simulink model "simc"  (R2020b)
settings: Solver=ode45  StartTime=0.0  StopTime=0.0005  RelTol=1e-3
values from neighbouring files (symbols this model uses):
  A = 8    [iraep.m]
  C = 9.5812e-5    (= 9.5812e-05)    [iraep.m]
  k = 1/(10^(-8.41/20))    (= 2.63329794368)    [iraep.m]
  ku1 = 0.7468    [iraep.m]
  L = 5.0498e-5    (= 5.0498e-05)    [iraep.m]
  Rs = 2.66    [iraep.m]    (also in simulare.m)
  U21 = 16    [iraep.m]
undefined symbols (not defined in the file or in its folder): den_pi, num_pi
settings Model: Creator=Alex  LastModifiedBy=Alex

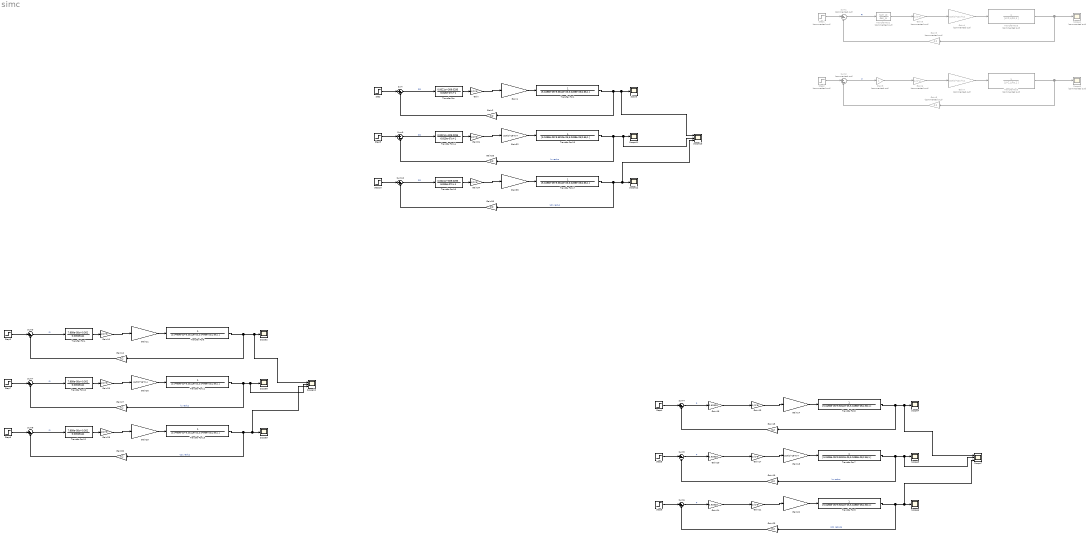
== system simc ==
  Gain{,10,13,17,21,25,28,31,34} (9 alike) : Gain  Gain=1/(2*8)
  Gain1 : Gain  Gain=sqrt(2)*16*0.7468
  Gain11 : Gain  Gain=sqrt(2)*16*0.7468
  Gain{2,12,15,19,23,27,30,33,36} (9 alike) : Gain  Gain=0.2
  Gain14 : Gain  Gain=sqrt(2)*16*0.7468
  Gain16 : Gain  Gain=2.63329
  Gain18 : Gain  Gain=sqrt(2)*16*0.4
  Gain20 : Gain  Gain=2.63329
  Gain22 : Gain  Gain=sqrt(2)*13*0.7468
  Gain24 : Gain  Gain=2.63329
  Gain26 : Gain  Gain=sqrt(2)*16*0.4
  Gain29 : Gain  Gain=sqrt(2)*13*0.7468
  Gain3 : Gain  Commented=on  Gain=1/(2*A)
  Gain32 : Gain  Gain=sqrt(2)*16*0.4
  Gain35 : Gain  Gain=sqrt(2)*13*0.7468
  Gain4 : Gain  Commented=on  Gain=sqrt(2)*U21*ku1
  Gain5 : Gain  Commented=on  Gain=0.2
  Gain6 : Gain  Commented=on  Gain=1/(2*A)
  Gain7 : Gain  Commented=on  Gain=sqrt(2)*U21*ku1
  Gain8 : Gain  Commented=on  Gain=0.2
  Gain9 : Gain  Commented=on  Gain=k
  Scope{,2,4..6,8..9,11..12} (9 alike) : Scope
  Scope1 : Scope  Commented=on
  Scope10 : Scope  NumInputPorts=3
  Scope13 : Scope  NumInputPorts=3
  Scope3 : Scope  Commented=on
  Scope7 : Scope  NumInputPorts=3
  Step{,3..10} (9 alike) : Step  Time=0  After=1.6  SampleTime=0
  Step1 : Step  Commented=on  Time=0  SampleTime=0
  Step2 : Step  Commented=on  Time=0  SampleTime=0
  Sum{,3..10} (9 alike) : Sum  Inputs=|+-
  Sum1 : Sum  Commented=on  Inputs=|+-
  Sum2 : Sum  Commented=on  Inputs=|+-
  Transfer Fcn : TransferFcn  Numerator="[0.0021  309.0295]"  Denominator=[6.815e-07 1]
  Transfer Fcn{1,6..9,11,13,15,17} (9 alike) : TransferFcn  Denominator=[5.0498e-05*9.5812e-05,5.0498e-05/2.66,1 ]
  Transfer Fcn10 : TransferFcn  Numerator="[7.895e-05  0.302]"  Denominator=[0.0002614 0]
  Transfer Fcn12 : TransferFcn  Numerator="[7.895e-05  0.302]"  Denominator=[0.0002614 0]
  Transfer Fcn14 : TransferFcn  Numerator="[0.0021  309.0295]"  Denominator=[6.815e-07 1]
  Transfer Fcn16 : TransferFcn  Numerator="[0.0021  309.0295]"  Denominator=[6.815e-07 1]
  Transfer Fcn2 : TransferFcn  Commented=on  Numerator=num_pi  Denominator=den_pi
  Transfer Fcn3 : TransferFcn  Commented=on  Denominator=[L*C,L/Rs,1 ]
  Transfer Fcn4 : TransferFcn  Numerator="[7.895e-05  0.302]"  Denominator=[0.0002614 0]
  Transfer Fcn5 : TransferFcn  Commented=on  Denominator=[L*C,L/Rs,1 ]
  wires:
  Step/1 -> Sum/1
  Sum/1 -> Transfer Fcn/1  "PD"
  Transfer Fcn/1 -> Gain/1
  Gain/1 -> Gain1/1
  Gain1/1 -> Transfer Fcn1/1
  Transfer Fcn1/1 -> Gain2/1, Scope13/1, Scope/1
  Gain2/1 -> Sum/2
  Gain5/1 -> Sum1/2
  Transfer Fcn3/1 -> Gain5/1, Scope1/1
  Gain4/1 -> Transfer Fcn3/1
  Gain3/1 -> Gain4/1
  Transfer Fcn2/1 -> Gain3/1
  Sum1/1 -> Transfer Fcn2/1  "PI"
  Step1/1 -> Sum1/1
  Step2/1 -> Sum2/1
  Sum2/1 -> Gain9/1  "P"
  Gain9/1 -> Gain6/1
  Gain6/1 -> Gain7/1
  Gain7/1 -> Transfer Fcn5/1
  Transfer Fcn5/1 -> Scope3/1, Gain8/1
  Gain8/1 -> Sum2/2
  Gain12/1 -> Sum3/2
  Transfer Fcn6/1 -> Scope10/1, Scope2/1, Gain12/1
  Gain11/1 -> Transfer Fcn6/1
  Gain10/1 -> Gain11/1
  Transfer Fcn4/1 -> Gain10/1
  Sum3/1 -> Transfer Fcn4/1  "PI"
  Step3/1 -> Sum3/1
  Step4/1 -> Sum4/1
  Sum4/1 -> Gain16/1  "P"
  Gain16/1 -> Gain13/1
  Gain13/1 -> Gain14/1
  Gain14/1 -> Transfer Fcn8/1
  Transfer Fcn8/1 -> Gain15/1, Scope7/1, Scope4/1
  Gain15/1 -> Sum4/2
  Gain19/1 -> Sum5/2
  Transfer Fcn7/1 -> Scope7/2, Scope5/1, Gain19/1  "ku redus"
  Gain18/1 -> Transfer Fcn7/1
  Gain17/1 -> Gain18/1
  Gain20/1 -> Gain17/1
  Sum5/1 -> Gain20/1  "P"
  Step5/1 -> Sum5/1
  Step6/1 -> Sum6/1
  Sum6/1 -> Gain24/1  "P"
  Gain24/1 -> Gain21/1
  Gain21/1 -> Gain22/1
  Gain22/1 -> Transfer Fcn9/1
  Transfer Fcn9/1 -> Gain23/1, Scope7/3, Scope6/1  "U21 redusa"
  Gain23/1 -> Sum6/2
  Step7/1 -> Sum7/1
  Sum7/1 -> Transfer Fcn10/1  "PI"
  Transfer Fcn10/1 -> Gain25/1
  Gain25/1 -> Gain26/1
  Gain26/1 -> Transfer Fcn11/1
  Transfer Fcn11/1 -> Gain27/1, Scope10/2, Scope8/1  "ku redus"
  Gain27/1 -> Sum7/2
  Gain30/1 -> Sum8/2
  Transfer Fcn13/1 -> Scope10/3, Scope9/1, Gain30/1  "U21 redus"
  Gain29/1 -> Transfer Fcn13/1
  Gain28/1 -> Gain29/1
  Transfer Fcn12/1 -> Gain28/1
  Sum8/1 -> Transfer Fcn12/1  "PI"
  Step8/1 -> Sum8/1
  Gain33/1 -> Sum9/2
  Transfer Fcn15/1 -> Scope13/2, Scope11/1, Gain33/1  "ku redus"
  Gain32/1 -> Transfer Fcn15/1
  Gain31/1 -> Gain32/1
  Transfer Fcn14/1 -> Gain31/1
  Sum9/1 -> Transfer Fcn14/1  "PD"
  Step9/1 -> Sum9/1
  Step10/1 -> Sum10/1
  Sum10/1 -> Transfer Fcn16/1  "PD"
  Transfer Fcn16/1 -> Gain34/1
  Gain34/1 -> Gain35/1
  Gain35/1 -> Transfer Fcn17/1
  Transfer Fcn17/1 -> Gain36/1, Scope13/3, Scope12/1  "U21 redus"
  Gain36/1 -> Sum10/2
